simulink model "PMSM_Alpha_beta"  (R2014b)
settings: Solver=ode23  StartTime=0.0  StopTime=500  FixedStep=1e-3  RelTol=1e-3
InitFcn:
  | R=0.875;
  | Ld=8.5e-3;
  | Lq=8.5e-3;
  | J=0.001; % Inertia of of the whole machine system is 2,5 times of motor inertia;
  | Ff=0.175;
  | 
  | L0=0.5*(Ld+Lq);
  | L2=0.5*(Ld-Lq);
settings Model: Creator=Visitor.user  LastModifiedBy=Lei
settings DataIOCC: SignalLoggingSaveFormat=ModelDataLogs
settings DebuggingCC: SaveWithParameterizedLinksMsg=none  UnderspecifiedInitializationDetection=Classic  MergeDetectMultiDrivingBlocksExec=none  MultiTaskCondExecSysMsg=none  FcnCallInpInsideContextMsg=UseLocalSettings
settings RTWCC: IncludeERTFirstTime=on
settings GRTTargetCC: CombineOutputUpdateFcns=off  GRTInterface=on

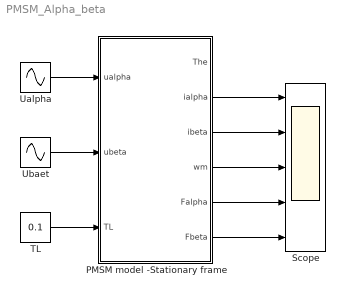
== system PMSM_Alpha_beta ==
  "PMSM model -Stationary frame " : Subsystem
  Scope : Scope  NumInputPorts=5
      settings: TimeRange=500  YMin=-10~-10~-0.05~-10~-10  YMax=15~10~0.2~10~10  SaveName=ScopeData2
  TL : Constant  Value=0.1
  Ualpha : Sin  Frequency=0.1  SampleTime=0
  Ubaet : Sin  Frequency=0.1  Phase=pi/2  SampleTime=0
  wires:
  Ualpha/1 -> "PMSM model -Stationary frame "/1(ualpha)
  Ubaet/1 -> "PMSM model -Stationary frame "/2(ubeta)
  "PMSM model -Stationary frame "/2(ialpha) -> Scope/1
  "PMSM model -Stationary frame "/3(ibeta) -> Scope/2
  "PMSM model -Stationary frame "/4(wm) -> Scope/3
  "PMSM model -Stationary frame "/5(Falpha) -> Scope/4
  "PMSM model -Stationary frame "/6(Fbeta) -> Scope/5
  TL/1 -> "PMSM model -Stationary frame "/3(TL)

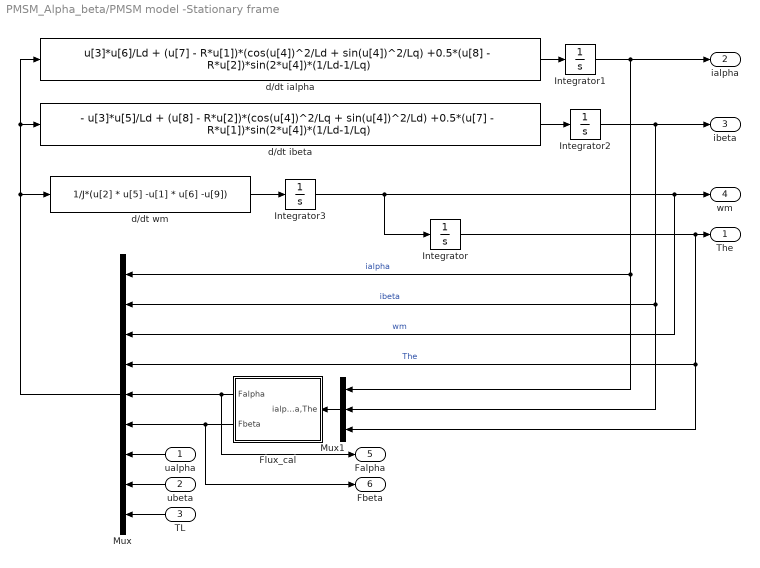
== system PMSM_Alpha_beta/PMSM model -Stationary frame  ==
  ualpha : Inport
  ubeta : Inport  Port=2
  TL : Inport  Port=3
  Flux_cal : Subsystem
  Integrator{,1..3} (4 alike) : Integrator
  Mux : Mux  Inputs=9
  Mux1 : Mux  Inputs=3
  d/dt ialpha : Fcn  Expr=u[3]*u[6]/Ld + (u[7] - R*u[1])*(cos(u[4])^2/Ld + sin(u[4])^2/Lq) +0.5*(u[8] - R*u[2])*sin(2*u[4])*(1/Ld-1/Lq)
  d/dt ibeta : Fcn  Expr=- u[3]*u[5]/Ld + (u[8] - R*u[2])*(cos(u[4])^2/Lq + sin(u[4])^2/Ld) +0.5*(u[7] - R*u[1])*sin(2*u[4])*(1/Ld-1/Lq)
  d/dt wm : Fcn  Expr=1/J*(u[2] * u[5] -u[1] * u[6] -u[9])
  The : Outport
  ialpha : Outport  Port=2
  ibeta : Outport  Port=3
  wm : Outport  Port=4
  Falpha : Outport  Port=5
  Fbeta : Outport  Port=6
  wires:
  d/dt ialpha/1 -> Integrator1/1
  Integrator1/1 -> Mux1/1, Mux/1, ialpha/1  "ialpha"
  Integrator2/1 -> ibeta/1, Mux/2, Mux1/2  "ibeta"
  d/dt wm/1 -> Integrator3/1
  Integrator3/1 -> wm/1, Mux/3, Integrator/1  "wm"
  Integrator/1 -> The/1, Mux1/3, Mux/4  "The"
  ualpha/1 -> Mux/7
  ubeta/1 -> Mux/8
  TL/1 -> Mux/9
  Mux/1 -> d/dt wm/1, d/dt ialpha/1, d/dt ibeta/1
  Flux_cal/1(Falpha) -> Falpha/1, Mux/5
  Flux_cal/2(Fbeta) -> Fbeta/1, Mux/6
  d/dt ibeta/1 -> Integrator2/1
  Mux1/1 -> Flux_cal/1(ialpha.ibeta,The)

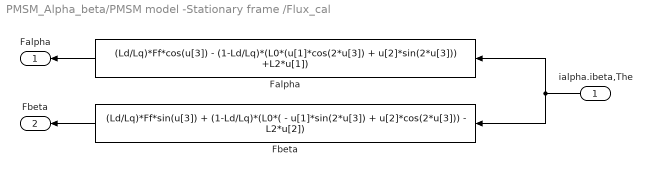
== system PMSM_Alpha_beta/PMSM model -Stationary frame /Flux_cal ==
  ialpha.ibeta,The : Inport
  " Falpha" : Fcn  Expr=(Ld/Lq)*Ff*cos(u[3]) - (1-Ld/Lq)*(L0*(u[1]*cos(2*u[3]) + u[2]*sin(2*u[3])) +L2*u[1])
  " Fbeta" : Fcn  Expr=(Ld/Lq)*Ff*sin(u[3]) + (1-Ld/Lq)*(L0*( - u[1]*sin(2*u[3]) + u[2]*cos(2*u[3])) - L2*u[2])
  Falpha : Outport
  Fbeta : Outport  Port=2
  wires:
  ialpha.ibeta,The/1 -> " Falpha"/1, " Fbeta"/1
  " Falpha"/1 -> Falpha/1
  " Fbeta"/1 -> Fbeta/1
